simulink model "n_trotinettes_crash_discret"  (Simulink 6.5)
settings: Solver=ode45  StartTime=0.0  StopTime=L  RelTol=1e-6
undefined symbols (not defined in the file or in its folder): Delta, DiscIntNeverNeededParam, K, Ka, Kd, Ki, Kv, L, M_ecart, N, Tau, Te
libraries: simulink_extras x1
settings Model: Creator=admin  LastModifiedBy=admin
settings DataIOCC: SignalLoggingName=sigsOut
settings DebuggingCC: SolverPrmCheckMsg=none  MultiTaskDSMMsg=warning  MultiTaskCondExecSysMsg=none  StrictBusMsg=None
settings HardwareCC: TargetUnknown=on
settings RTWCC: IncludeERTFirstTime=on

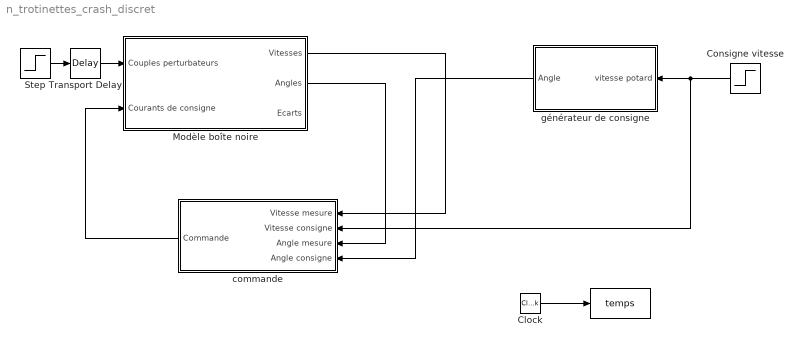
== system n_trotinettes_crash_discret ==
  " " : ToWorkspace  VariableName=temps  SampleTime=-1  SaveFormat=Array
  Clock : DigitalClock  SampleTime=Te
  Consigne vitesse : Step  Orientation=left  Time=L/2  Before=ones(N,1)*0.1  After=ones(N,1)  SampleTime=Te
  Modèle boîte noire : Subsystem
  Step : Step  Time=L*0.1  Before=zeros(N,1)  After=-ones(N,1)
  Transport Delay : TransportDelay  DelayTime=N-(1:N)
  commande : Subsystem  Orientation=left  TreatAsAtomicUnit=on
      settings: RTWSystemCode=Function  RTWFcnNameOpts=Use subsystem name  RTWFileNameOpts=Use subsystem name
  générateur de consigne : Subsystem  Orientation=left
  wires:
  Step/1 -> Transport Delay/1
  Consigne vitesse/1 -> commande/2(Vitesse consigne), générateur de consigne/1(vitesse potard)
  Modèle boîte noire/2(Angles) -> commande/3(Angle mesure)
  Clock/1 -> " "/1
  commande/1(Commande) -> Modèle boîte noire/2(Courants de consigne)
  Modèle boîte noire/1(Vitesses) -> commande/1(Vitesse mesure)
  générateur de consigne/1(Angle) -> commande/4(Angle consigne)
  Transport Delay/1 -> Modèle boîte noire/1(Couples perturbateurs)

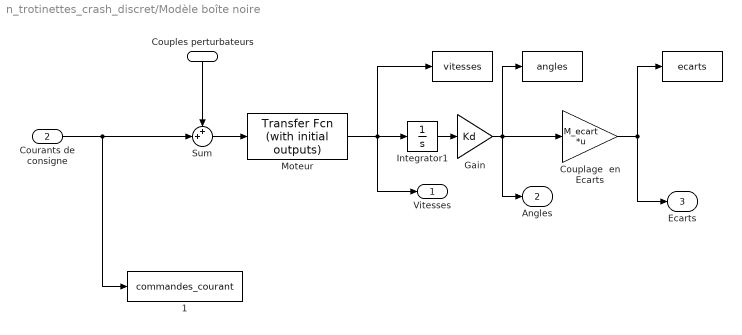
== system n_trotinettes_crash_discret/Modèle boîte noire ==
  Couples perturbateurs : Inport  Orientation=down
  Courants de consigne : Inport  Port=2
  " " : ToWorkspace  VariableName=vitesses  SampleTime=Te  SaveFormat=Array
  "  " : ToWorkspace  VariableName=angles  SampleTime=Te  SaveFormat=Array
  "   " : ToWorkspace  VariableName=ecarts  SampleTime=Te  SaveFormat=Array
  "   1" : ToWorkspace  VariableName=commandes_courant  SampleTime=-1  SaveFormat=Array
  Couplage  en Ecarts : Gain  Gain=M_ecart  Multiplication=Matrix(K*u)  SaturateOnIntegerOverflow=on
  Gain : Gain  Gain=Kd
  Integrator1 : Integrator  InitialCondition=927/Kd
  Moteur : simulink_extras/Additional Linear/Transfer Fcn (with initial outputs)  SystemSampleTime=-1  N=[K]  D="[Tau  1]"  Y0=0  U0=0
  Sum : Sum  Inputs=++|  SaturateOnIntegerOverflow=on
  Vitesses : Outport
  Angles : Outport  Port=2
  Ecarts : Outport  Port=3
  wires:
  Couplage  en Ecarts/1 -> Ecarts/1, "   "/1
  Courants de consigne/1 -> "   1"/1, Sum/2
  Couples perturbateurs/1 -> Sum/1
  Integrator1/1 -> Gain/1
  Sum/1 -> Moteur/1
  Moteur/1 -> Integrator1/1, " "/1, Vitesses/1
  Gain/1 -> Couplage  en Ecarts/1, Angles/1, "  "/1

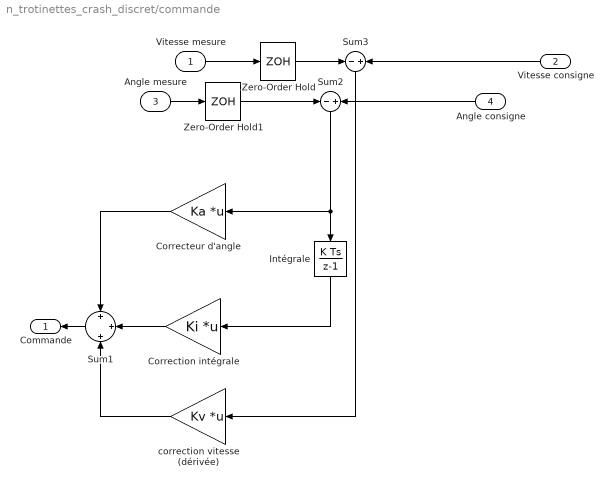
== system n_trotinettes_crash_discret/commande ==
  Vitesse mesure : Inport
  Vitesse consigne : Inport  Orientation=left  Port=2
  Angle mesure : Inport  Port=3
  Angle consigne : Inport  Orientation=left  Port=4
  Correcteur d'angle : Gain  Orientation=left  Gain=Ka  Multiplication=Matrix(K*u)  SaturateOnIntegerOverflow=on
  Correction intégrale : Gain  Orientation=left  Gain=Ki  Multiplication=Matrix(K*u)  SaturateOnIntegerOverflow=on
  Intégrale : DiscreteIntegrator  Orientation=down  InitialCondition=zeros(N,1)  SampleTime=Te  ICPrevOutput=DiscIntNeverNeededParam  ICPrevScaledInput=DiscIntNeverNeededParam
  Sum1 : Sum  Orientation=left  Inputs=+|+|+  SaturateOnIntegerOverflow=on
  Sum2 : Sum  Orientation=down  Inputs=-|+  SaturateOnIntegerOverflow=on
  Sum3 : Sum  Orientation=down  Inputs=-|+  SaturateOnIntegerOverflow=on
  Zero-Order Hold : ZeroOrderHold  SampleTime=Te
  Zero-Order Hold1 : ZeroOrderHold  SampleTime=Te
  correction vitesse (dérivée) : Gain  Orientation=left  Gain=Kv  Multiplication=Matrix(K*u)  SaturateOnIntegerOverflow=on
  Commande : Outport  Orientation=left
  wires:
  Sum2/1 -> Intégrale/1, Correcteur d'angle/1
  Correcteur d'angle/1 -> Sum1/1
  Sum3/1 -> correction vitesse (dérivée)/1
  Intégrale/1 -> Correction intégrale/1
  correction vitesse (dérivée)/1 -> Sum1/3
  Correction intégrale/1 -> Sum1/2
  Vitesse consigne/1 -> Sum3/2
  Angle consigne/1 -> Sum2/2
  Vitesse mesure/1 -> Zero-Order Hold/1
  Angle mesure/1 -> Zero-Order Hold1/1
  Sum1/1 -> Commande/1
  Zero-Order Hold/1 -> Sum3/1
  Zero-Order Hold1/1 -> Sum2/1

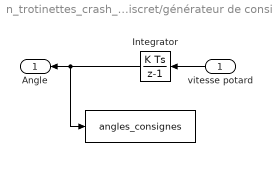
== system n_trotinettes_crash_discret/générateur de consigne ==
  vitesse potard : Inport  Orientation=left
  "  " : ToWorkspace  VariableName=angles_consignes  SampleTime=-1  SaveFormat=Array
  Integrator : DiscreteIntegrator  Orientation=left  InitialCondition=[0:N-1]'*Delta  SampleTime=Te  ICPrevOutput=DiscIntNeverNeededParam  ICPrevScaledInput=DiscIntNeverNeededParam
  Angle : Outport  Orientation=left
  wires:
  Integrator/1 -> "  "/1, Angle/1
  vitesse potard/1 -> Integrator/1
